simulink model "ODEModelLQR"  (R2024a)
settings: Solver=VariableStepAuto  StartTime=0.0  StopTime=simtime  RelTol=1e-9
values from neighbouring files (symbols this model uses):
  a = [0, 1; 0, (rho*A*C_D/m)*(v - alpha*u^beta)]    [tuneLQR_insilico.m]
  A = 4*3.14*0.02^2    (= 0.005024)    [tuneLQR_insilico.m]    (also in tunePID_empirical.m; tunePID_insilico.m)
  alpha = 0.1885    [tuneLQR_insilico.m]    (also in tunePID_empirical.m = 0.19; tunePID_insilico.m)
  b = [0; alpha*beta*rho*A*C_D/m*u^(beta - 1)*(alpha*u^beta - v)]    [tuneLQR_insilico.m]
  beta = 0.6272    [tuneLQR_insilico.m]    (also in tunePID_empirical.m = 0.63; tunePID_insilico.m)
  c = [1, 0]    [tuneLQR_insilico.m]
  C_D = 0.47    [tuneLQR_insilico.m]    (also in tunePID_empirical.m; tunePID_insilico.m)
  d = [0]    [tuneLQR_insilico.m]
  disturb_magnitude = -7.5    [tuneLQR_insilico.m]    (also in tunePID_insilico.m)
  disturb_time = 20    [tuneLQR_insilico.m]    (also in tunePID_insilico.m)
  g = 9.81    [tuneLQR_insilico.m]    (also in tunePID_empirical.m; tunePID_insilico.m)
  K = lqr(a,b,Q,1)    [tuneLQR_insilico.m]
  L = [100; 250000]    [tuneLQR_insilico.m]
  m = 0.00283    [tuneLQR_insilico.m]    (also in tunePID_empirical.m; tunePID_insilico.m)
  noise_sample_time = 0.05    [tuneLQR_insilico.m]    (also in tunePID_empirical.m; tunePID_insilico.m)
  rho = 1.225    [tuneLQR_insilico.m]    (also in tunePID_empirical.m; tunePID_insilico.m)
  steptime = 5    [tuneLQR_insilico.m]    (also in tunePID_empirical.m; tunePID_insilico.m)
  t_d = 0.5    [tuneLQR_insilico.m]    (also in tunePID_empirical.m; tunePID_insilico.m)
  tau = 0.05    [tuneLQR_insilico.m]    (also in tunePID_empirical.m = 0.01; tunePID_insilico.m)
  u_bar = (2*m*g/(rho*A*C_D*alpha^2))^(1/(2*beta))    (= 150.797926517)    [tuneLQR_insilico.m]
  z_0 = [0, 0]    [tuneLQR_insilico.m]    (also in tunePID_empirical.m = [0.2, 0]; tunePID_insilico.m)
  z_sp = out.simout(:,2)    [tuneLQR_insilico.m]    (also in tunePID_empirical.m = 0.4; tunePID_insilico.m)
libraries: simulink_extras x1, simulink x1
settings Model: Creator=twallema  LastModifiedBy=twallema
settings SolverCC: AlgebraicLoopSolver=TrustRegion
settings DebuggingCC: UnconnectedInputMsg=warning  UnconnectedOutputMsg=warning  UnconnectedLineMsg=warning
settings ModelReferenceCC: EnableRefExpFcnMdlSchedulingChecks=on
settings SFSimCC: CustomCodeUndefinedFunction=UseInterfaceOnly
settings RTWCC: GPUComputeCapability=3.5

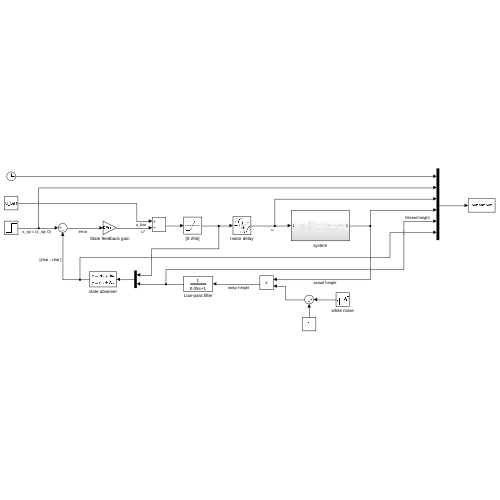
[thumbnail: Simulink's stored preview of the top-level diagram]
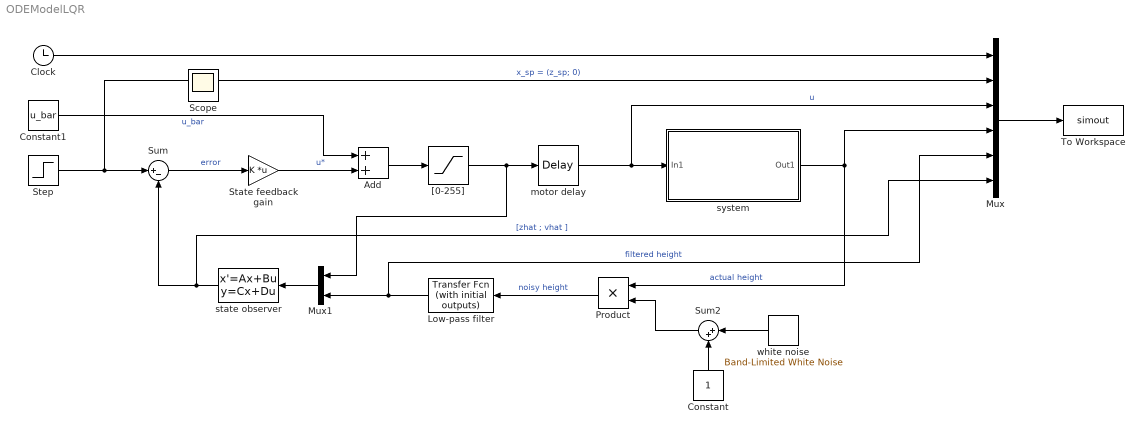
== system ODEModelLQR ==
  Add : Sum
  Clock : Clock
  Constant : Constant
  Constant1 : Constant  Value=u_bar
  Low-pass filter : simulink_extras/Additional Linear/Transfer Fcn (with initial outputs)  N=[1]  D="[tau  1]"  Y0=z_0(1)  U0=z_0(1)
  Mux : Mux  Inputs=6
  Mux1 : Mux  Inputs=2
  Product : Product
  State feedback gain : Gain  Gain=K  Multiplication=Matrix(K*u)
  Step : Step  Time=steptime  Before=[z_0(1); 0]  After=[z_sp; 0]  SampleTime=0
  Sum : Sum  Inputs=|+-
  Sum2 : Sum  Inputs=|++
  To Workspace : ToWorkspace  VariableName=simout  SampleTime=-1
  "[0-255]" : Saturate  UpperLimit=255  LowerLimit=0
  motor delay : TransportDelay  DelayTime=t_d  InitialOutput=u_bar
  state observer : StateSpace  A=(a-L*c)  B=[b-L*d L]  C=eye(2)  D=[0, 0; 0, 0]  InitialCondition=[z_0(1); 0]
  system : Subsystem
  white noise : simulink/Sources/Band-Limited White Noise  Cov=noise_power  Ts=noise_sample_time  seed=[23341]
  Scope : Scope
  wires:
  Mux/1 -> To Workspace/1
  system/1(Out1) -> Product/1, Mux/4  "actual height"
  "[0-255]"/1 -> Mux1/1, motor delay/1
  motor delay/1 -> Mux/3, system/1(In1)  "u"
  Add/1 -> "[0-255]"/1
  Step/1 -> Sum/1, Mux/2  "x_sp = (z_sp; 0)"
  Clock/1 -> Mux/1
  Product/1 -> Low-pass filter/1  "noisy height"
  white noise/1 -> Sum2/1
  Sum2/1 -> Product/2
  Constant/1 -> Sum2/2
  Low-pass filter/1 -> Mux1/2, Mux/5  "filtered height"
  Sum/1 -> State feedback gain/1  "error"
  state observer/1 -> Mux/6, Sum/2  "[zhat ; vhat ]"
  State feedback gain/1 -> Add/2  "u*"
  Constant1/1 -> Add/1  "u_bar"
  Mux1/1 -> state observer/1

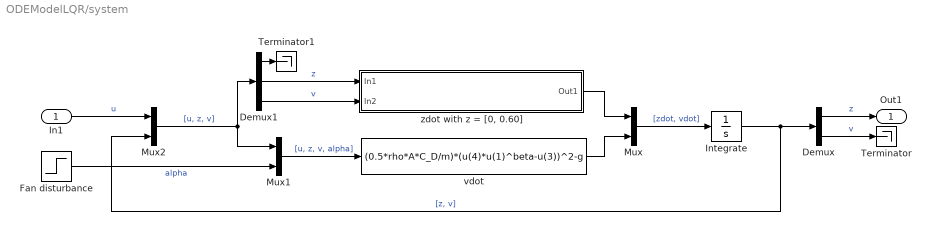
== system ODEModelLQR/system ==
  In1 : Inport
  Demux : Demux  Outputs=2
  Demux1 : Demux  Outputs=3
  Fan disturbance : Step  Time=disturb_time  Before=alpha  After=alpha*(1+disturb_magnitude/100)  SampleTime=0
  Integrate : Integrator  InitialCondition=z_0
  Mux : Mux  Inputs=2
  Mux1 : Mux  Inputs=2
  Mux2 : Mux  Inputs=2
  Terminator : Terminator
  Terminator1 : Terminator
  vdot : Fcn  Expr=(0.5*rho*A*C_D/m)*(u(4)*u(1)^beta-u(3))^2-g
  "zdot with z = [0, 0.60]" : Subsystem
  Out1 : Outport  VectorParamsAs1DForOutWhenUnconnected=off
  wires:
  vdot/1 -> Mux/2
  Mux2/1 -> Mux1/1, Demux1/1  "[u, z, v]"
  In1/1 -> Mux2/1  "u"
  Integrate/1 -> Demux/1, Mux2/2  "[z, v]"
  Mux/1 -> Integrate/1  "[zdot, vdot]"
  Demux1/1 -> Terminator1/1
  Demux1/3 -> "zdot with z = [0, 0.60]"/2(In2)  "v"
  Demux1/2 -> "zdot with z = [0, 0.60]"/1(In1)  "z"
  "zdot with z = [0, 0.60]"/1(Out1) -> Mux/1
  Mux1/1 -> vdot/1  "[u, z, v, alpha]"
  Fan disturbance/1 -> Mux1/2  "alpha"
  Demux/1 -> Out1/1  "z"
  Demux/2 -> Terminator/1  "v"

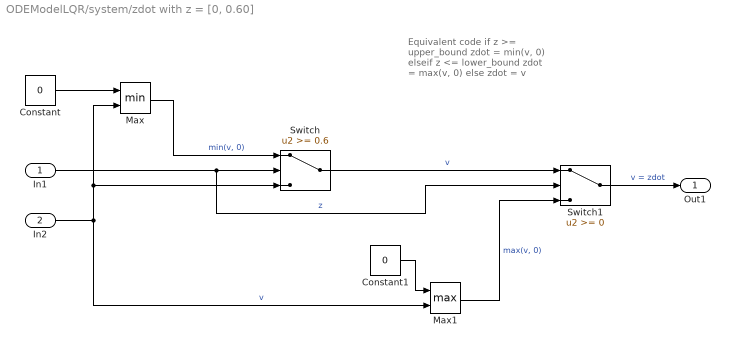
== system ODEModelLQR/system/zdot with z = [0, 0.60] ==
  note: Equivalent code
      |
      | if z >= upper_bound
      | zdot = min(v, 0)
      | elseif z <= lower_bound
      | zdot = max(v, 0)
      | else
      | zdot = v
  In1 : Inport
  In2 : Inport  Port=2
  Constant : Constant  Value=0
  Constant1 : Constant  Value=0
  Max : MinMax  Inputs=2
  Max1 : MinMax  Function=max  Inputs=2
  Switch : Switch  Threshold=0.6  SaturateOnIntegerOverflow=off  InputSameDT=off
  Switch1 : Switch  SaturateOnIntegerOverflow=off  InputSameDT=off
  Out1 : Outport
  wires:
  Max1/1 -> Switch1/3  "max(v, 0)"
  Constant/1 -> Max/1
  Constant1/1 -> Max1/1
  Switch/1 -> Switch1/1  "v"
  Max/1 -> Switch/1  "min(v, 0)"
  Switch1/1 -> Out1/1  "v = zdot"
  In1/1 -> Switch/2, Switch1/2  "z"
  In2/1 -> Max/2, Switch/3, Max1/2  "v"
